simulink model "StateFeedback"  (R2018b)
settings: Solver=VariableStepAuto  StartTime=0.0  StopTime=0.1  FixedStep=0.01  RelTol=1e-3
settings Model: Creator=Mr.Hallajiyan  LastModifiedBy=MJAHMADEE
settings SFSimCC: SimUseLocalCustomCode=off
settings RTWCC: RTWUseLocalCustomCode=off

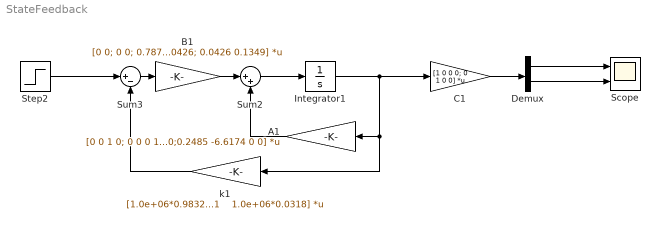
== system StateFeedback ==
  A1 : Gain  Gain=[0 0 1 0; 0 0 0 1; -0.4568 -0.6196 0 0;0.2485 -6.6174 0 0]  Multiplication=Matrix(K*u) (u vector)
  B1 : Gain  Gain=[0 0; 0 0; 0.7870 -0.0426; 0.0426 0.1349]  Multiplication=Matrix(K*u) (u vector)
  C1 : Gain  Gain=[1 0 0 0; 0 1 0 0]  Multiplication=Matrix(K*u) (u vector)
  Demux : Demux  Outputs=2
  Integrator1 : Integrator
  Scope : Scope  NumInputPorts=2
  Step2 : Step  Time=0  SampleTime=0.0001
  Sum2 : Sum  Inputs=|++
  Sum3 : Sum  Inputs=|+-
  k1 : Gain  Gain="[1.0e+06*0.9832    1.0e+06*0.1681    1.0e+06*0.0100    1.0e+06*0.0017;1.0e+06*-0.3105    1.0e+06*3.1048   1.0e+06*-0.0031    1.0e+06*0.0318]"  Multiplication=Matrix(K*u) (u vector)
  wires:
  Demux/2 -> Scope/2
  Demux/1 -> Scope/1
  Sum2/1 -> Integrator1/1
  Integrator1/1 -> C1/1, k1/1, A1/1
  C1/1 -> Demux/1
  B1/1 -> Sum2/1
  A1/1 -> Sum2/2
  k1/1 -> Sum3/2
  Sum3/1 -> B1/1
  Step2/1 -> Sum3/1
